simulink model "sistema_iniziale"  (R2019b)
settings: Solver=VariableStepAuto  StartTime=0.0  StopTime=10.0  RelTol=1e-3
undefined symbols (not defined in the file): den_G1, den_G2, num_G1, num_G2
settings Model: Creator=edoardo  LastModifiedBy=edoardo

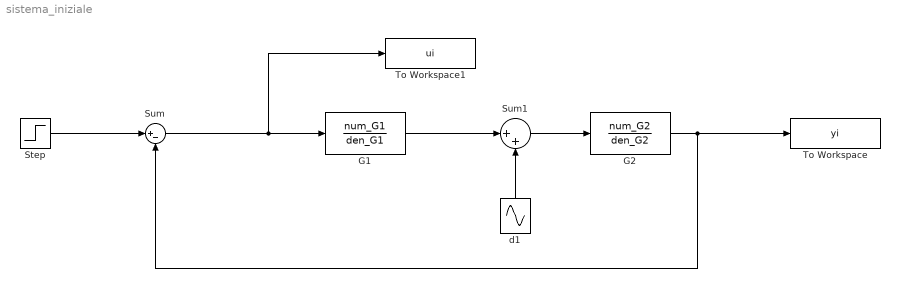
== system sistema_iniziale ==
  "G1 " : TransferFcn  Numerator=num_G1  Denominator=den_G1
  G2 : TransferFcn  Numerator=num_G2  Denominator=den_G2
  Step : Step  Time=0  After=1.5  SampleTime=0
  Sum : Sum  Inputs=|+-
  Sum1 : Sum  Inputs=|++
  To Workspace : ToWorkspace  VariableName=yi  SaveFormat=Timeseries  SampleTime=-1
  To Workspace1 : ToWorkspace  VariableName=ui  SaveFormat=Timeseries  SampleTime=-1
  d1 : Sin  Amplitude=3  SampleTime=0
  wires:
  Sum1/1 -> G2/1
  "G1 "/1 -> Sum1/1
  Step/1 -> Sum/1
  d1/1 -> Sum1/2
  G2/1 -> Sum/2, To Workspace/1
  Sum/1 -> To Workspace1/1, "G1 "/1
